simulink model "Watertank"  (R2023b)
settings: Solver=VariableStepAuto  StartTime=0.0  StopTime=200  RelTol=1e-3
undefined symbols (not defined in the file): DiscIntNeverNeededParam, TSRL
libraries: simulink x3, rllib x1
settings Model: Creator=Jan  LastModifiedBy=juliu
settings SolverCC: AlgebraicLoopSolver=TrustRegion
settings DebuggingCC: UnconnectedInputMsg=warning  UnconnectedOutputMsg=warning  UnconnectedLineMsg=warning
settings ModelReferenceCC: EnableRefExpFcnMdlSchedulingChecks=on
settings RTWCC: DLArmComputeVersion=19.05

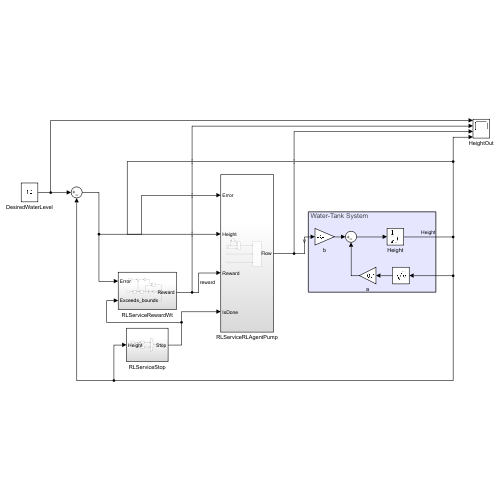
[thumbnail: Simulink's stored preview of the top-level diagram]
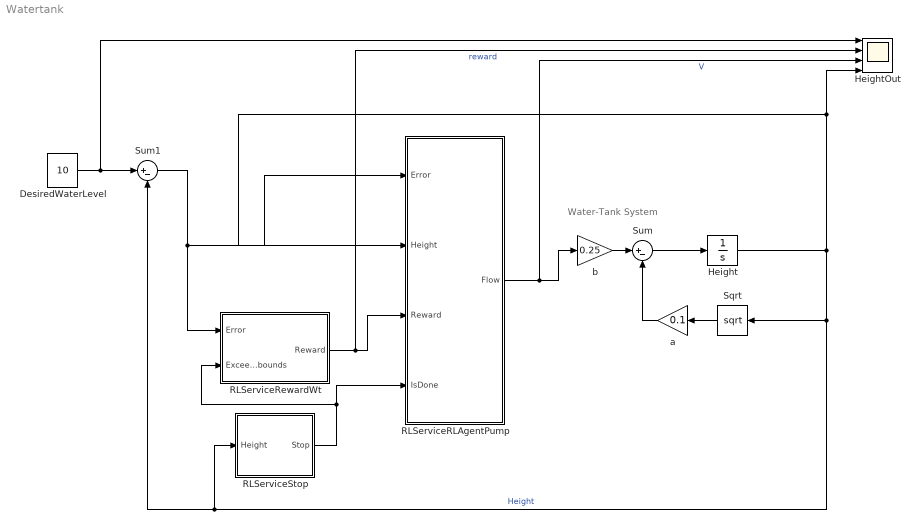
== system Watertank ==
  note: Water-Tank System
  DesiredWaterLevel : Constant  Value=10
  Height : Integrator  InitialCondition=3  LimitOutput=on  LowerSaturationLimit=0  ZeroCross=off
  HeightOut : Scope  NumInputPorts=4
  RLServiceRLAgentPump : Subsystem
  RLServiceRewardWt : Subsystem
  RLServiceStop : Subsystem
  Sqrt : Sqrt  OutputSignalType=real
  Sum : Sum  Inputs=|+-  SaturateOnIntegerOverflow=on
  Sum1 : Sum  Inputs=|+-  SaturateOnIntegerOverflow=on
  a : Gain  Gain=0.1  SaturateOnIntegerOverflow=on  OutDataTypeStr=Inherit: Same as input  ParamDataTypeStr=Inherit: Same as input
  b : Gain  Gain=0.25  SaturateOnIntegerOverflow=on  OutDataTypeStr=Inherit: Same as input  ParamDataTypeStr=Inherit: Same as input
  wires:
  Sqrt/1 -> a/1
  RLServiceRewardWt/1(Reward) -> HeightOut/2, RLServiceRLAgentPump/3(Reward)  "reward"
  RLServiceStop/1(Stop) -> RLServiceRLAgentPump/4(IsDone), RLServiceRewardWt/2(Exceeds_bounds)
  Sum1/1 -> RLServiceRewardWt/1(Error), RLServiceRLAgentPump/1(Error)
  Sum/1 -> Height/1
  Height/1 -> HeightOut/4, RLServiceRLAgentPump/2(Height), Sum1/2, RLServiceStop/1(Height), Sqrt/1  "Height"
  b/1 -> Sum/1
  RLServiceRLAgentPump/1(Flow) -> HeightOut/3, b/1  "V"
  a/1 -> Sum/2
  DesiredWaterLevel/1 -> HeightOut/1, Sum1/1

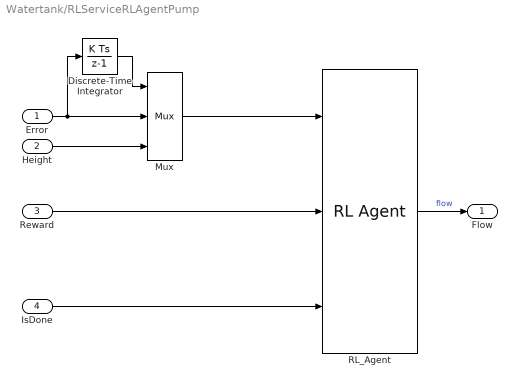
== system Watertank/RLServiceRLAgentPump ==
  Error : Inport
  Height : Inport  Port=2
  Reward : Inport  Port=3
  IsDone : Inport  Port=4
  Discrete-Time Integrator : DiscreteIntegrator  SampleTime=TSRL  ICPrevOutput=DiscIntNeverNeededParam  ICPrevScaledInput=DiscIntNeverNeededParam
  Mux : Mux  Inputs=3
  RL_Agent : rllib/RL Agent  Agent=agent  ExternalActionAsInput=off  ProvideCumRwd=off  TreatAsDirectFeedthrough=on
  Flow : Outport
  wires:
  RL_Agent/1 -> Flow/1  "flow"
  IsDone/1 -> RL_Agent/3
  Reward/1 -> RL_Agent/2
  Mux/1 -> RL_Agent/1
  Height/1 -> Mux/3
  Discrete-Time Integrator/1 -> Mux/1
  Error/1 -> Mux/2, Discrete-Time Integrator/1

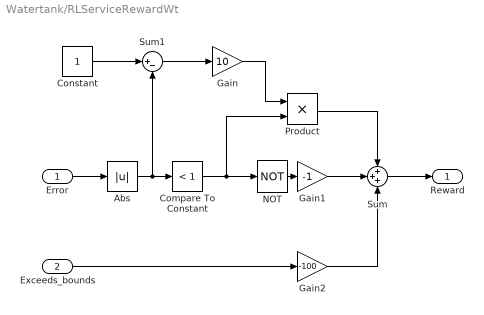
== system Watertank/RLServiceRewardWt ==
  Error : Inport
  Exceeds_bounds : Inport  Port=2
  Abs : Abs  SaturateOnIntegerOverflow=off
  Compare To Constant : simulink/Logic and Bit Operations/Compare To Constant  relop=<  const=1  OutDataTypeStr=boolean
  Constant : Constant
  Gain : Gain  Gain=10
  Gain1 : Gain  Gain=-1
  Gain2 : Gain  Gain=-100
  NOT : Logic  Operator=NOT  IconShape=distinctive  AllPortsSameDT=off  OutDataTypeStr=boolean
  Product : Product
  Sum : Sum  Inputs=+++  OutDataTypeStr=double
  Sum1 : Sum  Inputs=|+-
  Reward : Outport  VectorParamsAs1DForOutWhenUnconnected=off
  wires:
  Abs/1 -> Compare To Constant/1, Sum1/2
  Gain2/1 -> Sum/3
  Product/1 -> Sum/1
  Compare To Constant/1 -> Product/2, NOT/1
  Gain1/1 -> Sum/2
  Sum/1 -> Reward/1
  NOT/1 -> Gain1/1
  Exceeds_bounds/1 -> Gain2/1
  Error/1 -> Abs/1
  Constant/1 -> Sum1/1
  Sum1/1 -> Gain/1
  Gain/1 -> Product/1

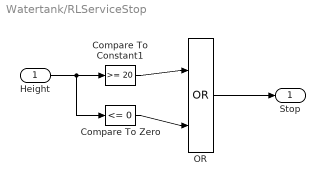
== system Watertank/RLServiceStop ==
  Height : Inport
  Compare To Constant1 : simulink/Logic and Bit Operations/Compare To Constant  relop=>=  const=20  OutDataTypeStr=boolean
  Compare To Zero : simulink/Logic and Bit Operations/Compare To Zero  relop=<=  OutDataTypeStr=boolean
  OR : Logic  Operator=OR  IconShape=distinctive  AllPortsSameDT=off  OutDataTypeStr=boolean
  Stop : Outport  VectorParamsAs1DForOutWhenUnconnected=off
  wires:
  Height/1 -> Compare To Zero/1, Compare To Constant1/1
  Compare To Zero/1 -> OR/2
  Compare To Constant1/1 -> OR/1
  OR/1 -> Stop/1
